simulink model "Battery_Pack_Thermal_Management"  (R2021b)
settings: Solver=ode23t  StartTime=0.0  StopTime=2400  MaxStep=0.05  RelTol=1e-3  AbsTol=1e-3
PreLoadFcn:
  | Battery_Pack_Thermal_Management_param
undefined symbols (not defined in the file): ambient, coolantTemp, R12, R23, R34, R45, R56, R67, R78
libraries: nesl_utility x35, fl_lib x10, batteryModule_lib x8, ee_lib x1
(part 1 of 2)
Description:
  | Battery Pack Thermal Management
  | 
  | Copyright 2020-2021 The MathWorks, Inc.
settings Model: Creator=vikrants  LastModifiedBy=smiller
settings SolverCC: AutoScaleAbsTol=off  AlgebraicLoopSolver=TrustRegion
settings DataIOCC: ReturnWorkspaceOutputs=off  SignalLoggingName=logsout_Battery_Pack_Thermal_Management
settings DebuggingCC: SymbolicDimsDataTypeCodeGenerationDiagnostic=none  SFMachineParentedDataDiag=warning
settings SFSimCC: CustomCodeUndefinedFunction=UseInterfaceOnly
settings SimscapeCC: SimscapeLogType=all  SimscapeLogSimulationStatistics=on  SimscapeLogName=simlog_Battery_Pack_Thermal_Management  SimscapeLogDataHistory=250000

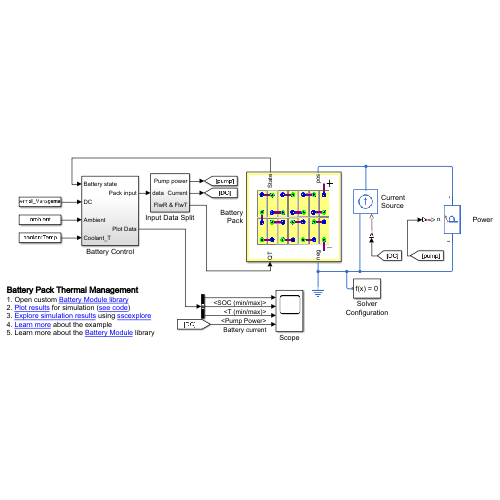
[thumbnail: Simulink's stored preview of the top-level diagram]
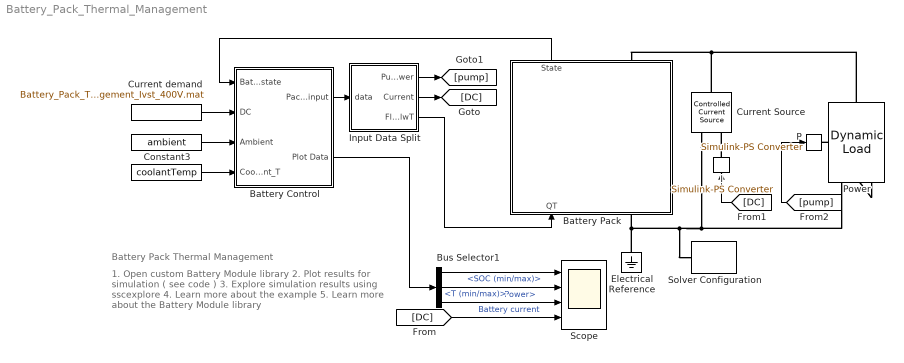
== system Battery_Pack_Thermal_Management ==
  note: 1. Open custom Battery Module library
      | 2. Plot results for simulation ( see code )
      | 3. Explore simulation results using sscexplore
      | 4. Learn more about the example
      | 5. Learn more about the Battery Module library
  note: Battery Pack Thermal Management
  " " : Constant  Value=coolantTemp
  Battery Pack : Subsystem
      mask Display: image('batteryPackIcon.png'); % Use "Edit Image" on toolstrip to change.
  Battery Control : Subsystem
  Bus Selector1 : BusSelector  OutputSignals=SOC (min/max),T (min/max),Pump Power
  Constant3 : Constant  Value=ambient
  Current Source : fl_lib/Electrical/Electrical Sources/Controlled Current Source
  Current demand : FromFile  FileName=Battery_Pack_Thermal_Management_Ivst_400V.mat  SampleTime=0
  Electrical Reference : fl_lib/Electrical/Electrical Elements/Electrical Reference
  I : nesl_utility/Simulink-PS Converter  PhysicalDomain=network_engine_domain  SubClassName=ps_input  LeftPortType=input  RightPortType=output  PseudoPeriodic=off  Frequencies=[]  NoiseDistribution=none  NoiseParameters=[]  Unit=A  AffineConversion=off  FilteringAndDerivatives=provide  SimscapeFilterOrder=1  InputFilterTimeConstant=0.001  UdotUserProvided=0
      settings: SourceProductName=Utilities
  Input Data Split : Subsystem
  P : nesl_utility/Simulink-PS Converter  PhysicalDomain=network_engine_domain  SubClassName=ps_input  LeftPortType=input  RightPortType=output  PseudoPeriodic=off  Frequencies=[]  NoiseDistribution=none  NoiseParameters=[]  Unit=J/s  AffineConversion=off  FilteringAndDerivatives=provide  SimscapeFilterOrder=1  InputFilterTimeConstant=0.001  UdotUserProvided=0
      settings: SourceProductName=Utilities
  Power : ee_lib/Passive/Dynamic Load  load_type=ee.enum.dc_ac.dc  min_supply_voltage=20 V  pow_min=1e-3 W  G_reverse=1e-6 S  deltaV=1e-3 V  f0=60 Hz  Vrms_min=200 V  Pmin=1e-3 W  enable_fault=simscape.enum.onoff.off  fault_action=simscape.enum.assert.action.none  t_fault=1 s  open_conductance=1e-4 S
      settings: SourceProductBaseCode=PS  InternalSimscapePortConfiguration="{\"Bottom\":[],\"Left\":[{\"id\":\"p\",\"label\":\"+\",\"type\":\"foundation.electrical.electrical\"}],\"Right\":[{\"id\":\"n\",\"label\":\"-\",\"type\":\"foundation.electrical.electrical\"}],\"Top\":[{\"id\":\"P\",\"label\":\"P\",\"type\":\"input\"}]}"
  Scope : Scope  NumInputPorts=4
  Solver Configuration : nesl_utility/Solver Configuration  PhysicalDomain=network_engine_domain  SubClassName=solver  LeftPortType=input  RightPortType=generic  Tones=[]  Harmonics=[]  SimulateNoise=off  Profile=off  UseLocalSampling=off  EnableSwitchedLinearOptims=on  FrequencyDomain=off  UseCCode=off  RelTol=0.001  AbsTol=1e-06  MinStep=1e-09  ToWorkspace=off  RevertToSquareIcSolve=off  NumHomotopyIterations=100  PhasorMode=off  PhasorModeNumHarmonics=1  DoDC=off  ResidualTolerance=1e-09  UseLocalSolver=off  LocalSolverChoice=NE_BACKWARD_EULER_ADVANCER  LocalSolverSampleTime=0.001  DoFixedCost=off  MaxNonlinIter=3  MaxModeIter=2  ComputeImpulses=off  ImpulseIterations=2  LinearAlgebra=auto  EquationFormulation=NE_TIME_EF  DelaysMemoryBudget=1024  AutomaticFiltering=on  FilteringTimeConstant=0.001  PartitionStorageMethod=AS_NEEDED  PartitionMemoryBudget=1024  PartitionMethod=ROBUST
      settings: SourceProductName=Utilities
  wires:
  Current demand/1 -> Battery Control/2(DC)
  Battery Pack/1(State) -> Battery Control/1(Battery state)
  Constant3/1 -> Battery Control/3(Ambient)
  Input Data Split/2(Current) -> [DC]
  Input Data Split/1(Pump power) -> [pump]
  [DC] -> Scope/4  "Battery current"
  Battery Control/1(Pack input) -> Input Data Split/1(data)
  Battery Control/2(Plot Data) -> Bus Selector1/1
  Bus Selector1/1 -> Scope/1  "<SOC (min/max)>"
  Bus Selector1/3 -> Scope/3  "<Pump Power>"
  Bus Selector1/2 -> Scope/2  "<T (min/max)>"
  Input Data Split/3(FlwR & FlwT) -> Battery Pack/1(QT)
  " "/1 -> Battery Control/4(Coolant_T)
  [DC] -> I/1
  [pump] -> P/1
  connections:
  Current Source/RConn2 -- Electrical Reference/LConn1 -- Battery Pack/LConn1 -- Solver Configuration/RConn1 -- Power/LConn1
  Current Source/LConn1 -- Power/RConn1 -- Battery Pack/RConn1
  Power/LConn2 -- P/RConn1
  I/RConn1 -- Current Source/RConn1

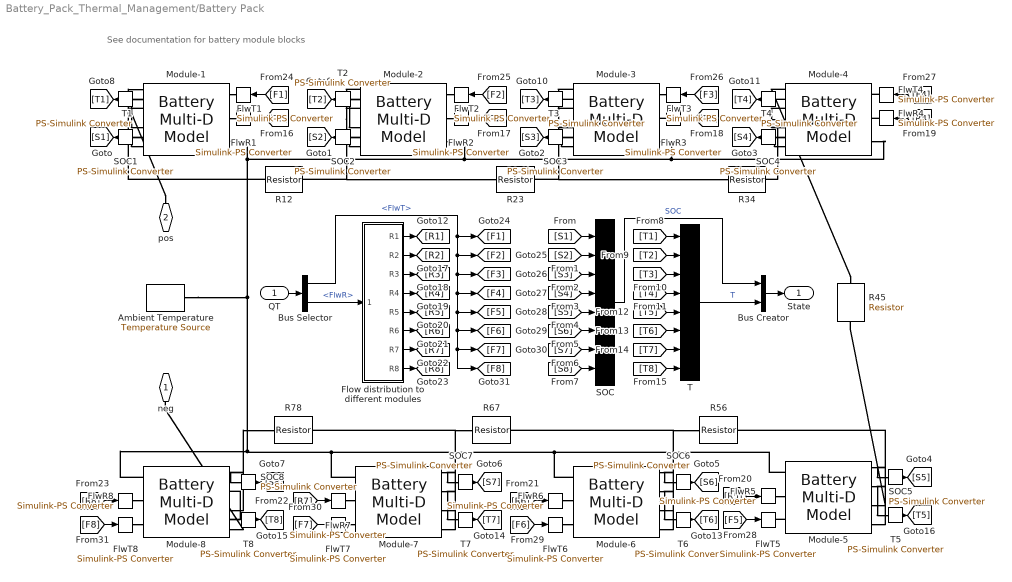
== system Battery_Pack_Thermal_Management/Battery Pack ==
  note: See documentation for battery module blocks
  QT : Inport
  Ambient Temperature : fl_lib/Thermal/Thermal Sources/Temperature Source  temperature=ambient K
  Bus Creator : BusCreator  Inputs=2
  Bus Selector : BusSelector  OutputSignals=FlwT,FlwR
  Flow distribution to different modules : Subsystem
  FlwR{1..8} (8 alike) : nesl_utility/Simulink-PS Converter  PhysicalDomain=network_engine_domain  SubClassName=ps_input  LeftPortType=input  RightPortType=output  PseudoPeriodic=off  Frequencies=[]  NoiseDistribution=none  NoiseParameters=[]  Unit=1  AffineConversion=off  FilteringAndDerivatives=provide  SimscapeFilterOrder=1  InputFilterTimeConstant=0.001  UdotUserProvided=0
      settings: SourceProductName=Utilities
  FlwT{1..8} (8 alike) : nesl_utility/Simulink-PS Converter  PhysicalDomain=network_engine_domain  SubClassName=ps_input  LeftPortType=input  RightPortType=output  PseudoPeriodic=off  Frequencies=[]  NoiseDistribution=none  NoiseParameters=[]  Unit=1  AffineConversion=off  FilteringAndDerivatives=provide  SimscapeFilterOrder=1  InputFilterTimeConstant=0.001  UdotUserProvided=0
      settings: SourceProductName=Utilities
  Module-1 : batteryModule_lib/Battery Multi-D Model  modelComplexity=batteryModule.batteryAbstractionLevel.grouped  LUTpointsTemp=T_vec K  cellAHvector=AH_vec hr*A  LUTpointsSOC=SOC_vec  V0_mat=V0_mat V  prm_dir=ee.enum.battery.prm_dir.noCurrentDirectionality  R0_mat=R0_mat Ohm  R0_dis_mat=[.03, .015, .002; .04, .017, .008; .039, .012, .006; .027, .013, .021] Ohm  R0_ch_mat=[.03, .015, .002; .04, .017, .008; .039, .012, .006; .027, .013, .021] Ohm  prm_leak=ee.enum.battery.prm_leak.disabled  Rleak_vec=[8000, 7000, 6000] Ohm  extrapolation_option=ee.enum.extrapolation.nearest  prm_dyn=ee.enum.battery.prm_dyn.rc2  R1_mat=R1_mat Ohm  tau1_mat=Tau1_mat s  R2_mat=R2_mat Ohm  tau2_mat=Tau2_mat s  R3_mat=[.014, .382, .407; .028, .006, .007; .014, .007, .006; .333, .956, .912] Ohm  tau3_mat=[1, 44, 5644; 11, 24, 506; 2, 14, 330; 3310, 13419, 30216] s  R4_mat=[.014, .382, .407; .028, .006, .007; .014, .007, .006; .333, .956, .912] Ohm  tau4_mat=[1, 44, 5644; 11, 24, 506; 2, 14, 330; 3310, 13419, 30216] s  R5_mat=[.014, .382, .407; .028, .006, .007; .014, .007, .006; .333, .956, .912] Ohm  tau5_mat=[1, 44, 5644; 11, 24, 506; 2, 14, 330; 3310, 13419, 30216] s  prm_fade=ee.enum.battery.prm_fade.equations  N0=Ndisc  dV0=delV0  dR0=delR0  dAH=delAH0  dRleak=0  dR1=delR1  dR2=delR2  dR3=0  dR4=0  dR5=0  N0vec=[100, 200, 300]  Tfadevec=[298.15, 323.15] K  dV0vec=[0, 0, 0]  dR0vec=[0, 0, 0]  dAHvec=[0, 0, 0]  dRleakvec=[0, 0, 0]  dR1vec=[0, 0, 0]  dR2vec=[0, 0, 0]  dR3vec=[0, 0, 0]  dR4vec=[0, 0, 0]  dR5vec=[0, 0, 0]  dV0mat=[0, 0; 0, 0; 0, 0]  dR0mat=[0, 0; 0, 0; 0, 0]  dAHmat=[0, 0; 0, 0; 0, 0]  dRleakmat=[0, 0; 0, 0; 0, 0]  dR1mat=[0, 0; 0, 0; 0, 0]  dR2mat=[0, 0; 0, 0; 0, 0]  dR3mat=[0, 0; 0, 0; 0, 0]  dR4mat=[0, 0; 0, 0; 0, 0]  dR5mat=[0, 0; 0, 0; 0, 0]  cellThermalMass=MdotCp J/K  cellThermalCond=K_cell W/(m*K)  cellThermalCond_inPlane=20 W/(m*K)  Ns=Ns1  Np=Np1  cellTypeSelection=batteryModule.batteryTypeSelection.pouch  cellHeight=cell_H m  cellWidth=cell_W m  cellThickness=cell_T m  cellDiameter=0.018 m  cellCylinLine=3  moduleExternalR=Rext1 Ohm  moduleCellBalancing=batteryModule.batteryCellBalancing.none  passiveShuntR=50 Ohm  passiveSWclosedR=0.01 Ohm  passiveSWopenCond=1e-8 1/Ohm  passiveSWthreshold=0.5  thermalManagement=batteryModule.batteryCoolingSystem.thermalPort  cellHeatTrCoeff=h_cell W/(m^2 * K)  thermal_moduleBottom=batteryModule.batteryThermalPortSelection.thermalLUT  htc_bottom=1 W/(m^2 * K)  moduleCooling_b=Q1 W/K  LUTpointsFlowrate_b=Flowrate_vec kg/s  LUTpointsTemp_b=T_vec K  thermal_moduleTop=batteryModule.batteryThermalPortSelection.convectionBC  htc_top=h_cell W/(m^2 * K)  moduleCooling_t=zeros(3, 6, 10) W/K  LUTpointsFlowrate_t=[.01, .02, .03, .04, .05, .06] kg/s  LUTpointsTemp_t=[273.15, 298.15, 323.15] K  thermal_moduleRight=batteryModule.batteryThermalPortSelection.convectionBC  htc_right=h_cell W/(m^2 * K)  moduleCooling_r=zeros(3, 6, 10) W/K  LUTpointsFlowrate_r=[.01, .02, .03, .04, .05, .06] kg/s  LUTpointsTemp_r=[273.15, 298.15, 323.15] K  thermal_moduleLeft=batteryModule.batteryThermalPortSelection.convectionBC  htc_left=h_cell W/(m^2 * K)  moduleCooling_l=zeros(3, 6, 10) W/K  LUTpointsFlowrate_l=[.01, .02, .03, .04, .05, .06] kg/s  LUTpointsTemp_l=[273.15, 298.15, 323.15] K  thermal_modulePos=batteryModule.batteryThermalPortSelection.convectionBC  htc_pos=h_cell W/(m^2 * K)  moduleCooling_p=zeros(3, 6, 10) W/K  LUTpointsFlowrate_p=[.01, .02, .03, .04, .05, .06] kg/s  LUTpointsTemp_p=[273.15, 298.15, 323.15] K  thermal_moduleNeg=batteryModule.batteryThermalPortSelection.convectionBC  htc_neg=h_cell W/(m^2 * K)  moduleCooling_n=zeros(3, 6, 10) W/K  LUTpointsFlowrate_n=[.01, .02, .03, .04, .05, .06] kg/s  LUTpointsTemp_n=[273.15, 298.15, 323.15] K  moduleExtHeat=extQ1 W  cellTemp=iniT1 K  cellSOC=iniSOC1  moduleCellAHpercentVar=iniAH1  moduleCellLeakPercentVar=ones(1, 10)  moduleCellR0PercentVar=iniR01
      settings: SourceProductName=Some kind of I/O error occurred when accessing database . (disk I/O error)  InternalSimscapePortConfiguration="{\"Bottom\":[],\"Left\":[{\"id\":\"outputCellSOC\",\"label\":\"SOC\",\"type\":\"output\"},{\"id\":\"outputCellTemp\",\"label\":\"Temp\",\"type\":\"output\"}],\"Right\":[{\"id\":\"H\",\"label\":\"Amb\",\"type\":\"foundation.thermal.thermal\"},{\"id\":\"frac_b\",\"label\":\"FlwR\",\"type\":\"input\"},{\"id\":\"delT_b\",\"label\":\"FlwT\",\"type\":\"input\"}],\"Top\":[{\"id\":\"p\",\"label\":\"pos\",\"type\":\"foundation.electrical.electrical\"},{\"id\":\"n\",\"label\":\"neg\",\"type\":\"foundation.electrical.electrical\"}]}"
  Module-2 : batteryModule_lib/Battery Multi-D Model  modelComplexity=batteryModule.batteryAbstractionLevel.grouped  LUTpointsTemp=T_vec K  cellAHvector=AH_vec hr*A  LUTpointsSOC=SOC_vec  V0_mat=V0_mat V  prm_dir=ee.enum.battery.prm_dir.noCurrentDirectionality  R0_mat=R0_mat Ohm  R0_dis_mat=[.03, .015, .002; .04, .017, .008; .039, .012, .006; .027, .013, .021] Ohm  R0_ch_mat=[.03, .015, .002; .04, .017, .008; .039, .012, .006; .027, .013, .021] Ohm  prm_leak=ee.enum.battery.prm_leak.disabled  Rleak_vec=[8000, 7000, 6000] Ohm  extrapolation_option=ee.enum.extrapolation.nearest  prm_dyn=ee.enum.battery.prm_dyn.rc2  R1_mat=R1_mat Ohm  tau1_mat=Tau1_mat s  R2_mat=R2_mat Ohm  tau2_mat=Tau2_mat s  R3_mat=[.014, .382, .407; .028, .006, .007; .014, .007, .006; .333, .956, .912] Ohm  tau3_mat=[1, 44, 5644; 11, 24, 506; 2, 14, 330; 3310, 13419, 30216] s  R4_mat=[.014, .382, .407; .028, .006, .007; .014, .007, .006; .333, .956, .912] Ohm  tau4_mat=[1, 44, 5644; 11, 24, 506; 2, 14, 330; 3310, 13419, 30216] s  R5_mat=[.014, .382, .407; .028, .006, .007; .014, .007, .006; .333, .956, .912] Ohm  tau5_mat=[1, 44, 5644; 11, 24, 506; 2, 14, 330; 3310, 13419, 30216] s  prm_fade=ee.enum.battery.prm_fade.equations  N0=Ndisc  dV0=delV0  dR0=delR0  dAH=delAH0  dRleak=0  dR1=delR1  dR2=delR2  dR3=0  dR4=0  dR5=0  N0vec=[100, 200, 300]  Tfadevec=[298.15, 323.15] K  dV0vec=[0, 0, 0]  dR0vec=[0, 0, 0]  dAHvec=[0, 0, 0]  dRleakvec=[0, 0, 0]  dR1vec=[0, 0, 0]  dR2vec=[0, 0, 0]  dR3vec=[0, 0, 0]  dR4vec=[0, 0, 0]  dR5vec=[0, 0, 0]  dV0mat=[0, 0; 0, 0; 0, 0]  dR0mat=[0, 0; 0, 0; 0, 0]  dAHmat=[0, 0; 0, 0; 0, 0]  dRleakmat=[0, 0; 0, 0; 0, 0]  dR1mat=[0, 0; 0, 0; 0, 0]  dR2mat=[0, 0; 0, 0; 0, 0]  dR3mat=[0, 0; 0, 0; 0, 0]  dR4mat=[0, 0; 0, 0; 0, 0]  dR5mat=[0, 0; 0, 0; 0, 0]  cellThermalMass=MdotCp J/K  cellThermalCond=K_cell W/(m*K)  cellThermalCond_inPlane=20 W/(m*K)  Ns=Ns2  Np=Np2  cellTypeSelection=batteryModule.batteryTypeSelection.pouch  cellHeight=cell_H m  cellWidth=cell_W m  cellThickness=cell_T m  cellDiameter=0.018 m  cellCylinLine=3  moduleExternalR=Rext2 Ohm  moduleCellBalancing=batteryModule.batteryCellBalancing.none  passiveShuntR=50 Ohm  passiveSWclosedR=0.01 Ohm  passiveSWopenCond=1e-8 1/Ohm  passiveSWthreshold=0.5  thermalManagement=batteryModule.batteryCoolingSystem.thermalPort  cellHeatTrCoeff=h_cell W/(m^2 * K)  thermal_moduleBottom=batteryModule.batteryThermalPortSelection.thermalLUT  htc_bottom=1 W/(m^2 * K)  moduleCooling_b=Q2 W/K  LUTpointsFlowrate_b=Flowrate_vec kg/s  LUTpointsTemp_b=T_vec K  thermal_moduleTop=batteryModule.batteryThermalPortSelection.convectionBC  htc_top=h_cell W/(m^2 * K)  moduleCooling_t=zeros(3, 6, 10) W/K  LUTpointsFlowrate_t=[.01, .02, .03, .04, .05, .06] kg/s  LUTpointsTemp_t=[273.15, 298.15, 323.15] K  thermal_moduleRight=batteryModule.batteryThermalPortSelection.convectionBC  htc_right=h_cell W/(m^2 * K)  moduleCooling_r=zeros(3, 6, 10) W/K  LUTpointsFlowrate_r=[.01, .02, .03, .04, .05, .06] kg/s  LUTpointsTemp_r=[273.15, 298.15, 323.15] K  thermal_moduleLeft=batteryModule.batteryThermalPortSelection.convectionBC  htc_left=h_cell W/(m^2 * K)  moduleCooling_l=zeros(3, 6, 10) W/K  LUTpointsFlowrate_l=[.01, .02, .03, .04, .05, .06] kg/s  LUTpointsTemp_l=[273.15, 298.15, 323.15] K  thermal_modulePos=batteryModule.batteryThermalPortSelection.convectionBC  htc_pos=h_cell W/(m^2 * K)  moduleCooling_p=zeros(3, 6, 10) W/K  LUTpointsFlowrate_p=[.01, .02, .03, .04, .05, .06] kg/s  LUTpointsTemp_p=[273.15, 298.15, 323.15] K  thermal_moduleNeg=batteryModule.batteryThermalPortSelection.convectionBC  htc_neg=h_cell W/(m^2 * K)  moduleCooling_n=zeros(3, 6, 10) W/K  LUTpointsFlowrate_n=[.01, .02, .03, .04, .05, .06] kg/s  LUTpointsTemp_n=[273.15, 298.15, 323.15] K  moduleExtHeat=extQ2 W  cellTemp=iniT2 K  cellSOC=iniSOC2  moduleCellAHpercentVar=iniAH2  moduleCellLeakPercentVar=ones(1, 10)  moduleCellR0PercentVar=iniR02
      settings: SourceProductName=Some kind of I/O error occurred when accessing database . (disk I/O error)  InternalSimscapePortConfiguration="{\"Bottom\":[],\"Left\":[{\"id\":\"outputCellSOC\",\"label\":\"SOC\",\"type\":\"output\"},{\"id\":\"outputCellTemp\",\"label\":\"Temp\",\"type\":\"output\"}],\"Right\":[{\"id\":\"H\",\"label\":\"Amb\",\"type\":\"foundation.thermal.thermal\"},{\"id\":\"frac_b\",\"label\":\"FlwR\",\"type\":\"input\"},{\"id\":\"delT_b\",\"label\":\"FlwT\",\"type\":\"input\"}],\"Top\":[{\"id\":\"p\",\"label\":\"pos\",\"type\":\"foundation.electrical.electrical\"},{\"id\":\"n\",\"label\":\"neg\",\"type\":\"foundation.electrical.electrical\"}]}"
  Module-3 : batteryModule_lib/Battery Multi-D Model  modelComplexity=batteryModule.batteryAbstractionLevel.grouped  LUTpointsTemp=T_vec K  cellAHvector=AH_vec hr*A  LUTpointsSOC=SOC_vec  V0_mat=V0_mat V  prm_dir=ee.enum.battery.prm_dir.noCurrentDirectionality  R0_mat=R0_mat Ohm  R0_dis_mat=[.03, .015, .002; .04, .017, .008; .039, .012, .006; .027, .013, .021] Ohm  R0_ch_mat=[.03, .015, .002; .04, .017, .008; .039, .012, .006; .027, .013, .021] Ohm  prm_leak=ee.enum.battery.prm_leak.disabled  Rleak_vec=[8000, 7000, 6000] Ohm  extrapolation_option=ee.enum.extrapolation.nearest  prm_dyn=ee.enum.battery.prm_dyn.rc2  R1_mat=R1_mat Ohm  tau1_mat=Tau1_mat s  R2_mat=R2_mat Ohm  tau2_mat=Tau2_mat s  R3_mat=[.014, .382, .407; .028, .006, .007; .014, .007, .006; .333, .956, .912] Ohm  tau3_mat=[1, 44, 5644; 11, 24, 506; 2, 14, 330; 3310, 13419, 30216] s  R4_mat=[.014, .382, .407; .028, .006, .007; .014, .007, .006; .333, .956, .912] Ohm  tau4_mat=[1, 44, 5644; 11, 24, 506; 2, 14, 330; 3310, 13419, 30216] s  R5_mat=[.014, .382, .407; .028, .006, .007; .014, .007, .006; .333, .956, .912] Ohm  tau5_mat=[1, 44, 5644; 11, 24, 506; 2, 14, 330; 3310, 13419, 30216] s  prm_fade=ee.enum.battery.prm_fade.equations  N0=Ndisc  dV0=delV0  dR0=delR0  dAH=delAH0  dRleak=0  dR1=delR1  dR2=delR2  dR3=0  dR4=0  dR5=0  N0vec=[100, 200, 300]  Tfadevec=[298.15, 323.15] K  dV0vec=[0, 0, 0]  dR0vec=[0, 0, 0]  dAHvec=[0, 0, 0]  dRleakvec=[0, 0, 0]  dR1vec=[0, 0, 0]  dR2vec=[0, 0, 0]  dR3vec=[0, 0, 0]  dR4vec=[0, 0, 0]  dR5vec=[0, 0, 0]  dV0mat=[0, 0; 0, 0; 0, 0]  dR0mat=[0, 0; 0, 0; 0, 0]  dAHmat=[0, 0; 0, 0; 0, 0]  dRleakmat=[0, 0; 0, 0; 0, 0]  dR1mat=[0, 0; 0, 0; 0, 0]  dR2mat=[0, 0; 0, 0; 0, 0]  dR3mat=[0, 0; 0, 0; 0, 0]  dR4mat=[0, 0; 0, 0; 0, 0]  dR5mat=[0, 0; 0, 0; 0, 0]  cellThermalMass=MdotCp J/K  cellThermalCond=K_cell W/(m*K)  cellThermalCond_inPlane=20 W/(m*K)  Ns=Ns3  Np=Np3  cellTypeSelection=batteryModule.batteryTypeSelection.pouch  cellHeight=cell_H m  cellWidth=cell_W m  cellThickness=cell_T m  cellDiameter=0.018 m  cellCylinLine=3  moduleExternalR=Rext3 Ohm  moduleCellBalancing=batteryModule.batteryCellBalancing.none  passiveShuntR=50 Ohm  passiveSWclosedR=0.01 Ohm  passiveSWopenCond=1e-8 1/Ohm  passiveSWthreshold=0.5  thermalManagement=batteryModule.batteryCoolingSystem.thermalPort  cellHeatTrCoeff=h_cell W/(m^2 * K)  thermal_moduleBottom=batteryModule.batteryThermalPortSelection.thermalLUT  htc_bottom=1 W/(m^2 * K)  moduleCooling_b=Q3 W/K  LUTpointsFlowrate_b=Flowrate_vec kg/s  LUTpointsTemp_b=T_vec K  thermal_moduleTop=batteryModule.batteryThermalPortSelection.convectionBC  htc_top=h_cell W/(m^2 * K)  moduleCooling_t=zeros(3, 6, 10) W/K  LUTpointsFlowrate_t=[.01, .02, .03, .04, .05, .06] kg/s  LUTpointsTemp_t=[273.15, 298.15, 323.15] K  thermal_moduleRight=batteryModule.batteryThermalPortSelection.convectionBC  htc_right=h_cell W/(m^2 * K)  moduleCooling_r=zeros(3, 6, 10) W/K  LUTpointsFlowrate_r=[.01, .02, .03, .04, .05, .06] kg/s  LUTpointsTemp_r=[273.15, 298.15, 323.15] K  thermal_moduleLeft=batteryModule.batteryThermalPortSelection.convectionBC  htc_left=h_cell W/(m^2 * K)  moduleCooling_l=zeros(3, 6, 10) W/K  LUTpointsFlowrate_l=[.01, .02, .03, .04, .05, .06] kg/s  LUTpointsTemp_l=[273.15, 298.15, 323.15] K  thermal_modulePos=batteryModule.batteryThermalPortSelection.convectionBC  htc_pos=h_cell W/(m^2 * K)  moduleCooling_p=zeros(3, 6, 10) W/K  LUTpointsFlowrate_p=[.01, .02, .03, .04, .05, .06] kg/s  LUTpointsTemp_p=[273.15, 298.15, 323.15] K  thermal_moduleNeg=batteryModule.batteryThermalPortSelection.convectionBC  htc_neg=h_cell W/(m^2 * K)  moduleCooling_n=zeros(3, 6, 10) W/K  LUTpointsFlowrate_n=[.01, .02, .03, .04, .05, .06] kg/s  LUTpointsTemp_n=[273.15, 298.15, 323.15] K  moduleExtHeat=extQ3 W  cellTemp=iniT3 K  cellSOC=iniSOC3  moduleCellAHpercentVar=iniAH3  moduleCellLeakPercentVar=ones(1, 10)  moduleCellR0PercentVar=iniR03
      settings: SourceProductName=Some kind of I/O error occurred when accessing database . (disk I/O error)  InternalSimscapePortConfiguration="{\"Bottom\":[],\"Left\":[{\"id\":\"outputCellSOC\",\"label\":\"SOC\",\"type\":\"output\"},{\"id\":\"outputCellTemp\",\"label\":\"Temp\",\"type\":\"output\"}],\"Right\":[{\"id\":\"H\",\"label\":\"Amb\",\"type\":\"foundation.thermal.thermal\"},{\"id\":\"frac_b\",\"label\":\"FlwR\",\"type\":\"input\"},{\"id\":\"delT_b\",\"label\":\"FlwT\",\"type\":\"input\"}],\"Top\":[{\"id\":\"p\",\"label\":\"pos\",\"type\":\"foundation.electrical.electrical\"},{\"id\":\"n\",\"label\":\"neg\",\"type\":\"foundation.electrical.electrical\"}]}"
  Module-4 : batteryModule_lib/Battery Multi-D Model  modelComplexity=batteryModule.batteryAbstractionLevel.grouped  LUTpointsTemp=T_vec K  cellAHvector=AH_vec hr*A  LUTpointsSOC=SOC_vec  V0_mat=V0_mat V  prm_dir=ee.enum.battery.prm_dir.noCurrentDirectionality  R0_mat=R0_mat Ohm  R0_dis_mat=[.03, .015, .002; .04, .017, .008; .039, .012, .006; .027, .013, .021] Ohm  R0_ch_mat=[.03, .015, .002; .04, .017, .008; .039, .012, .006; .027, .013, .021] Ohm  prm_leak=ee.enum.battery.prm_leak.disabled  Rleak_vec=[8000, 7000, 6000] Ohm  extrapolation_option=ee.enum.extrapolation.nearest  prm_dyn=ee.enum.battery.prm_dyn.rc2  R1_mat=R1_mat Ohm  tau1_mat=Tau1_mat s  R2_mat=R2_mat Ohm  tau2_mat=Tau2_mat s  R3_mat=[.014, .382, .407; .028, .006, .007; .014, .007, .006; .333, .956, .912] Ohm  tau3_mat=[1, 44, 5644; 11, 24, 506; 2, 14, 330; 3310, 13419, 30216] s  R4_mat=[.014, .382, .407; .028, .006, .007; .014, .007, .006; .333, .956, .912] Ohm  tau4_mat=[1, 44, 5644; 11, 24, 506; 2, 14, 330; 3310, 13419, 30216] s  R5_mat=[.014, .382, .407; .028, .006, .007; .014, .007, .006; .333, .956, .912] Ohm  tau5_mat=[1, 44, 5644; 11, 24, 506; 2, 14, 330; 3310, 13419, 30216] s  prm_fade=ee.enum.battery.prm_fade.equations  N0=Ndisc  dV0=delV0  dR0=delR0  dAH=delAH0  dRleak=0  dR1=delR1  dR2=delR2  dR3=0  dR4=0  dR5=0  N0vec=[100, 200, 300]  Tfadevec=[298.15, 323.15] K  dV0vec=[0, 0, 0]  dR0vec=[0, 0, 0]  dAHvec=[0, 0, 0]  dRleakvec=[0, 0, 0]  dR1vec=[0, 0, 0]  dR2vec=[0, 0, 0]  dR3vec=[0, 0, 0]  dR4vec=[0, 0, 0]  dR5vec=[0, 0, 0]  dV0mat=[0, 0; 0, 0; 0, 0]  dR0mat=[0, 0; 0, 0; 0, 0]  dAHmat=[0, 0; 0, 0; 0, 0]  dRleakmat=[0, 0; 0, 0; 0, 0]  dR1mat=[0, 0; 0, 0; 0, 0]  dR2mat=[0, 0; 0, 0; 0, 0]  dR3mat=[0, 0; 0, 0; 0, 0]  dR4mat=[0, 0; 0, 0; 0, 0]  dR5mat=[0, 0; 0, 0; 0, 0]  cellThermalMass=MdotCp J/K  cellThermalCond=K_cell W/(m*K)  cellThermalCond_inPlane=20 W/(m*K)  Ns=Ns4  Np=Np4  cellTypeSelection=batteryModule.batteryTypeSelection.pouch  cellHeight=cell_H m  cellWidth=cell_W m  cellThickness=cell_T m  cellDiameter=0.018 m  cellCylinLine=3  moduleExternalR=Rext4 Ohm  moduleCellBalancing=batteryModule.batteryCellBalancing.none  passiveShuntR=50 Ohm  passiveSWclosedR=0.01 Ohm  passiveSWopenCond=1e-8 1/Ohm  passiveSWthreshold=0.5  thermalManagement=batteryModule.batteryCoolingSystem.thermalPort  cellHeatTrCoeff=h_cell W/(m^2 * K)  thermal_moduleBottom=batteryModule.batteryThermalPortSelection.thermalLUT  htc_bottom=1 W/(m^2 * K)  moduleCooling_b=Q4 W/K  LUTpointsFlowrate_b=Flowrate_vec kg/s  LUTpointsTemp_b=T_vec K  thermal_moduleTop=batteryModule.batteryThermalPortSelection.convectionBC  htc_top=h_cell W/(m^2 * K)  moduleCooling_t=zeros(3, 6, 10) W/K  LUTpointsFlowrate_t=[.01, .02, .03, .04, .05, .06] kg/s  LUTpointsTemp_t=[273.15, 298.15, 323.15] K  thermal_moduleRight=batteryModule.batteryThermalPortSelection.convectionBC  htc_right=h_cell W/(m^2 * K)  moduleCooling_r=zeros(3, 6, 10) W/K  LUTpointsFlowrate_r=[.01, .02, .03, .04, .05, .06] kg/s  LUTpointsTemp_r=[273.15, 298.15, 323.15] K  thermal_moduleLeft=batteryModule.batteryThermalPortSelection.convectionBC  htc_left=h_cell W/(m^2 * K)  moduleCooling_l=zeros(3, 6, 10) W/K  LUTpointsFlowrate_l=[.01, .02, .03, .04, .05, .06] kg/s  LUTpointsTemp_l=[273.15, 298.15, 323.15] K  thermal_modulePos=batteryModule.batteryThermalPortSelection.convectionBC  htc_pos=h_cell W/(m^2 * K)  moduleCooling_p=zeros(3, 6, 10) W/K  LUTpointsFlowrate_p=[.01, .02, .03, .04, .05, .06] kg/s  LUTpointsTemp_p=[273.15, 298.15, 323.15] K  thermal_moduleNeg=batteryModule.batteryThermalPortSelection.convectionBC  htc_neg=h_cell W/(m^2 * K)  moduleCooling_n=zeros(3, 6, 10) W/K  LUTpointsFlowrate_n=[.01, .02, .03, .04, .05, .06] kg/s  LUTpointsTemp_n=[273.15, 298.15, 323.15] K  moduleExtHeat=extQ4 W  cellTemp=iniT4 K  cellSOC=iniSOC4  moduleCellAHpercentVar=iniAH4  moduleCellLeakPercentVar=ones(1, 10)  moduleCellR0PercentVar=iniR04
      settings: SourceProductName=Some kind of I/O error occurred when accessing database . (disk I/O error)  InternalSimscapePortConfiguration="{\"Bottom\":[],\"Left\":[{\"id\":\"outputCellSOC\",\"label\":\"SOC\",\"type\":\"output\"},{\"id\":\"outputCellTemp\",\"label\":\"Temp\",\"type\":\"output\"}],\"Right\":[{\"id\":\"H\",\"label\":\"Amb\",\"type\":\"foundation.thermal.thermal\"},{\"id\":\"frac_b\",\"label\":\"FlwR\",\"type\":\"input\"},{\"id\":\"delT_b\",\"label\":\"FlwT\",\"type\":\"input\"}],\"Top\":[{\"id\":\"p\",\"label\":\"pos\",\"type\":\"foundation.electrical.electrical\"},{\"id\":\"n\",\"label\":\"neg\",\"type\":\"foundation.electrical.electrical\"}]}"
  Module-5 : batteryModule_lib/Battery Multi-D Model  modelComplexity=batteryModule.batteryAbstractionLevel.grouped  LUTpointsTemp=T_vec K  cellAHvector=AH_vec hr*A  LUTpointsSOC=SOC_vec  V0_mat=V0_mat V  prm_dir=ee.enum.battery.prm_dir.noCurrentDirectionality  R0_mat=R0_mat Ohm  R0_dis_mat=[.03, .015, .002; .04, .017, .008; .039, .012, .006; .027, .013, .021] Ohm  R0_ch_mat=[.03, .015, .002; .04, .017, .008; .039, .012, .006; .027, .013, .021] Ohm  prm_leak=ee.enum.battery.prm_leak.disabled  Rleak_vec=[8000, 7000, 6000] Ohm  extrapolation_option=ee.enum.extrapolation.nearest  prm_dyn=ee.enum.battery.prm_dyn.rc2  R1_mat=R1_mat Ohm  tau1_mat=Tau1_mat s  R2_mat=R2_mat Ohm  tau2_mat=Tau2_mat s  R3_mat=[.014, .382, .407; .028, .006, .007; .014, .007, .006; .333, .956, .912] Ohm  tau3_mat=[1, 44, 5644; 11, 24, 506; 2, 14, 330; 3310, 13419, 30216] s  R4_mat=[.014, .382, .407; .028, .006, .007; .014, .007, .006; .333, .956, .912] Ohm  tau4_mat=[1, 44, 5644; 11, 24, 506; 2, 14, 330; 3310, 13419, 30216] s  R5_mat=[.014, .382, .407; .028, .006, .007; .014, .007, .006; .333, .956, .912] Ohm  tau5_mat=[1, 44, 5644; 11, 24, 506; 2, 14, 330; 3310, 13419, 30216] s  prm_fade=ee.enum.battery.prm_fade.equations  N0=Ndisc  dV0=delV0  dR0=delR0  dAH=delAH0  dRleak=0  dR1=delR1  dR2=delR2  dR3=0  dR4=0  dR5=0  N0vec=[100, 200, 300]  Tfadevec=[298.15, 323.15] K  dV0vec=[0, 0, 0]  dR0vec=[0, 0, 0]  dAHvec=[0, 0, 0]  dRleakvec=[0, 0, 0]  dR1vec=[0, 0, 0]  dR2vec=[0, 0, 0]  dR3vec=[0, 0, 0]  dR4vec=[0, 0, 0]  dR5vec=[0, 0, 0]  dV0mat=[0, 0; 0, 0; 0, 0]  dR0mat=[0, 0; 0, 0; 0, 0]  dAHmat=[0, 0; 0, 0; 0, 0]  dRleakmat=[0, 0; 0, 0; 0, 0]  dR1mat=[0, 0; 0, 0; 0, 0]  dR2mat=[0, 0; 0, 0; 0, 0]  dR3mat=[0, 0; 0, 0; 0, 0]  dR4mat=[0, 0; 0, 0; 0, 0]  dR5mat=[0, 0; 0, 0; 0, 0]  cellThermalMass=MdotCp J/K  cellThermalCond=K_cell W/(m*K)  cellThermalCond_inPlane=20 W/(m*K)  Ns=Ns5  Np=Np5  cellTypeSelection=batteryModule.batteryTypeSelection.pouch  cellHeight=cell_H m  cellWidth=cell_W m  cellThickness=cell_T m  cellDiameter=0.018 m  cellCylinLine=3  moduleExternalR=Rext5 Ohm  moduleCellBalancing=batteryModule.batteryCellBalancing.none  passiveShuntR=50 Ohm  passiveSWclosedR=0.01 Ohm  passiveSWopenCond=1e-8 1/Ohm  passiveSWthreshold=0.5  thermalManagement=batteryModule.batteryCoolingSystem.thermalPort  cellHeatTrCoeff=h_cell W/(m^2 * K)  thermal_moduleBottom=batteryModule.batteryThermalPortSelection.thermalLUT  htc_bottom=1 W/(m^2 * K)  moduleCooling_b=Q5 W/K  LUTpointsFlowrate_b=Flowrate_vec kg/s  LUTpointsTemp_b=T_vec K  thermal_moduleTop=batteryModule.batteryThermalPortSelection.convectionBC  htc_top=h_cell W/(m^2 * K)  moduleCooling_t=zeros(3, 6, 10) W/K  LUTpointsFlowrate_t=[.01, .02, .03, .04, .05, .06] kg/s  LUTpointsTemp_t=[273.15, 298.15, 323.15] K  thermal_moduleRight=batteryModule.batteryThermalPortSelection.convectionBC  htc_right=h_cell W/(m^2 * K)  moduleCooling_r=zeros(3, 6, 10) W/K  LUTpointsFlowrate_r=[.01, .02, .03, .04, .05, .06] kg/s  LUTpointsTemp_r=[273.15, 298.15, 323.15] K  thermal_moduleLeft=batteryModule.batteryThermalPortSelection.convectionBC  htc_left=h_cell W/(m^2 * K)  moduleCooling_l=zeros(3, 6, 10) W/K  LUTpointsFlowrate_l=[.01, .02, .03, .04, .05, .06] kg/s  LUTpointsTemp_l=[273.15, 298.15, 323.15] K  thermal_modulePos=batteryModule.batteryThermalPortSelection.convectionBC  htc_pos=h_cell W/(m^2 * K)  moduleCooling_p=zeros(3, 6, 10) W/K  LUTpointsFlowrate_p=[.01, .02, .03, .04, .05, .06] kg/s  LUTpointsTemp_p=[273.15, 298.15, 323.15] K  thermal_moduleNeg=batteryModule.batteryThermalPortSelection.convectionBC  htc_neg=h_cell W/(m^2 * K)  moduleCooling_n=zeros(3, 6, 10) W/K  LUTpointsFlowrate_n=[.01, .02, .03, .04, .05, .06] kg/s  LUTpointsTemp_n=[273.15, 298.15, 323.15] K  moduleExtHeat=extQ5 W  cellTemp=iniT5 K  cellSOC=iniSOC5  moduleCellAHpercentVar=iniAH5  moduleCellLeakPercentVar=ones(1, 10)  moduleCellR0PercentVar=iniR05
      settings: SourceProductName=Some kind of I/O error occurred when accessing database . (disk I/O error)  InternalSimscapePortConfiguration="{\"Bottom\":[],\"Left\":[{\"id\":\"outputCellSOC\",\"label\":\"SOC\",\"type\":\"output\"},{\"id\":\"outputCellTemp\",\"label\":\"Temp\",\"type\":\"output\"}],\"Right\":[{\"id\":\"H\",\"label\":\"Amb\",\"type\":\"foundation.thermal.thermal\"},{\"id\":\"frac_b\",\"label\":\"FlwR\",\"type\":\"input\"},{\"id\":\"delT_b\",\"label\":\"FlwT\",\"type\":\"input\"}],\"Top\":[{\"id\":\"p\",\"label\":\"pos\",\"type\":\"foundation.electrical.electrical\"},{\"id\":\"n\",\"label\":\"neg\",\"type\":\"foundation.electrical.electrical\"}]}"
  Module-6 : batteryModule_lib/Battery Multi-D Model  modelComplexity=batteryModule.batteryAbstractionLevel.grouped  LUTpointsTemp=T_vec K  cellAHvector=AH_vec hr*A  LUTpointsSOC=SOC_vec  V0_mat=V0_mat V  prm_dir=ee.enum.battery.prm_dir.noCurrentDirectionality  R0_mat=R0_mat Ohm  R0_dis_mat=[.03, .015, .002; .04, .017, .008; .039, .012, .006; .027, .013, .021] Ohm  R0_ch_mat=[.03, .015, .002; .04, .017, .008; .039, .012, .006; .027, .013, .021] Ohm  prm_leak=ee.enum.battery.prm_leak.disabled  Rleak_vec=[8000, 7000, 6000] Ohm  extrapolation_option=ee.enum.extrapolation.nearest  prm_dyn=ee.enum.battery.prm_dyn.rc2  R1_mat=R1_mat Ohm  tau1_mat=Tau1_mat s  R2_mat=R2_mat Ohm  tau2_mat=Tau2_mat s  R3_mat=[.014, .382, .407; .028, .006, .007; .014, .007, .006; .333, .956, .912] Ohm  tau3_mat=[1, 44, 5644; 11, 24, 506; 2, 14, 330; 3310, 13419, 30216] s  R4_mat=[.014, .382, .407; .028, .006, .007; .014, .007, .006; .333, .956, .912] Ohm  tau4_mat=[1, 44, 5644; 11, 24, 506; 2, 14, 330; 3310, 13419, 30216] s  R5_mat=[.014, .382, .407; .028, .006, .007; .014, .007, .006; .333, .956, .912] Ohm  tau5_mat=[1, 44, 5644; 11, 24, 506; 2, 14, 330; 3310, 13419, 30216] s  prm_fade=ee.enum.battery.prm_fade.equations  N0=Ndisc  dV0=delV0  dR0=delR0  dAH=delAH0  dRleak=0  dR1=delR1  dR2=delR2  dR3=0  dR4=0  dR5=0  N0vec=[100, 200, 300]  Tfadevec=[298.15, 323.15] K  dV0vec=[0, 0, 0]  dR0vec=[0, 0, 0]  dAHvec=[0, 0, 0]  dRleakvec=[0, 0, 0]  dR1vec=[0, 0, 0]  dR2vec=[0, 0, 0]  dR3vec=[0, 0, 0]  dR4vec=[0, 0, 0]  dR5vec=[0, 0, 0]  dV0mat=[0, 0; 0, 0; 0, 0]  dR0mat=[0, 0; 0, 0; 0, 0]  dAHmat=[0, 0; 0, 0; 0, 0]  dRleakmat=[0, 0; 0, 0; 0, 0]  dR1mat=[0, 0; 0, 0; 0, 0]  dR2mat=[0, 0; 0, 0; 0, 0]  dR3mat=[0, 0; 0, 0; 0, 0]  dR4mat=[0, 0; 0, 0; 0, 0]  dR5mat=[0, 0; 0, 0; 0, 0]  cellThermalMass=MdotCp J/K  cellThermalCond=K_cell W/(m*K)  cellThermalCond_inPlane=20 W/(m*K)  Ns=Ns6  Np=Np6  cellTypeSelection=batteryModule.batteryTypeSelection.pouch  cellHeight=cell_H m  cellWidth=cell_W m  cellThickness=cell_T m  cellDiameter=0.018 m  cellCylinLine=3  moduleExternalR=Rext6 Ohm  moduleCellBalancing=batteryModule.batteryCellBalancing.none  passiveShuntR=50 Ohm  passiveSWclosedR=0.01 Ohm  passiveSWopenCond=1e-8 1/Ohm  passiveSWthreshold=0.5  thermalManagement=batteryModule.batteryCoolingSystem.thermalPort  cellHeatTrCoeff=h_cell W/(m^2 * K)  thermal_moduleBottom=batteryModule.batteryThermalPortSelection.thermalLUT  htc_bottom=1 W/(m^2 * K)  moduleCooling_b=Q6 W/K  LUTpointsFlowrate_b=Flowrate_vec kg/s  LUTpointsTemp_b=T_vec K  thermal_moduleTop=batteryModule.batteryThermalPortSelection.convectionBC  htc_top=h_cell W/(m^2 * K)  moduleCooling_t=zeros(3, 6, 10) W/K  LUTpointsFlowrate_t=[.01, .02, .03, .04, .05, .06] kg/s  LUTpointsTemp_t=[273.15, 298.15, 323.15] K  thermal_moduleRight=batteryModule.batteryThermalPortSelection.convectionBC  htc_right=h_cell W/(m^2 * K)  moduleCooling_r=zeros(3, 6, 10) W/K  LUTpointsFlowrate_r=[.01, .02, .03, .04, .05, .06] kg/s  LUTpointsTemp_r=[273.15, 298.15, 323.15] K  thermal_moduleLeft=batteryModule.batteryThermalPortSelection.convectionBC  htc_left=h_cell W/(m^2 * K)  moduleCooling_l=zeros(3, 6, 10) W/K  LUTpointsFlowrate_l=[.01, .02, .03, .04, .05, .06] kg/s  LUTpointsTemp_l=[273.15, 298.15, 323.15] K  thermal_modulePos=batteryModule.batteryThermalPortSelection.convectionBC  htc_pos=h_cell W/(m^2 * K)  moduleCooling_p=zeros(3, 6, 10) W/K  LUTpointsFlowrate_p=[.01, .02, .03, .04, .05, .06] kg/s  LUTpointsTemp_p=[273.15, 298.15, 323.15] K  thermal_moduleNeg=batteryModule.batteryThermalPortSelection.convectionBC  htc_neg=h_cell W/(m^2 * K)  moduleCooling_n=zeros(3, 6, 10) W/K  LUTpointsFlowrate_n=[.01, .02, .03, .04, .05, .06] kg/s  LUTpointsTemp_n=[273.15, 298.15, 323.15] K  moduleExtHeat=extQ6 W  cellTemp=iniT6 K  cellSOC=iniSOC6  moduleCellAHpercentVar=iniAH6  moduleCellLeakPercentVar=ones(1, 10)  moduleCellR0PercentVar=iniR06
      settings: SourceProductName=Some kind of I/O error occurred when accessing database . (disk I/O error)  InternalSimscapePortConfiguration="{\"Bottom\":[],\"Left\":[{\"id\":\"outputCellSOC\",\"label\":\"SOC\",\"type\":\"output\"},{\"id\":\"outputCellTemp\",\"label\":\"Temp\",\"type\":\"output\"}],\"Right\":[{\"id\":\"H\",\"label\":\"Amb\",\"type\":\"foundation.thermal.thermal\"},{\"id\":\"frac_b\",\"label\":\"FlwR\",\"type\":\"input\"},{\"id\":\"delT_b\",\"label\":\"FlwT\",\"type\":\"input\"}],\"Top\":[{\"id\":\"p\",\"label\":\"pos\",\"type\":\"foundation.electrical.electrical\"},{\"id\":\"n\",\"label\":\"neg\",\"type\":\"foundation.electrical.electrical\"}]}"
  Module-7 : batteryModule_lib/Battery Multi-D Model  modelComplexity=batteryModule.batteryAbstractionLevel.grouped  LUTpointsTemp=T_vec K  cellAHvector=AH_vec hr*A  LUTpointsSOC=SOC_vec  V0_mat=V0_mat V  prm_dir=ee.enum.battery.prm_dir.noCurrentDirectionality  R0_mat=R0_mat Ohm  R0_dis_mat=[.03, .015, .002; .04, .017, .008; .039, .012, .006; .027, .013, .021] Ohm  R0_ch_mat=[.03, .015, .002; .04, .017, .008; .039, .012, .006; .027, .013, .021] Ohm  prm_leak=ee.enum.battery.prm_leak.disabled  Rleak_vec=[8000, 7000, 6000] Ohm  extrapolation_option=ee.enum.extrapolation.nearest  prm_dyn=ee.enum.battery.prm_dyn.rc2  R1_mat=R1_mat Ohm  tau1_mat=Tau1_mat s  R2_mat=R2_mat Ohm  tau2_mat=Tau2_mat s  R3_mat=[.014, .382, .407; .028, .006, .007; .014, .007, .006; .333, .956, .912] Ohm  tau3_mat=[1, 44, 5644; 11, 24, 506; 2, 14, 330; 3310, 13419, 30216] s  R4_mat=[.014, .382, .407; .028, .006, .007; .014, .007, .006; .333, .956, .912] Ohm  tau4_mat=[1, 44, 5644; 11, 24, 506; 2, 14, 330; 3310, 13419, 30216] s  R5_mat=[.014, .382, .407; .028, .006, .007; .014, .007, .006; .333, .956, .912] Ohm  tau5_mat=[1, 44, 5644; 11, 24, 506; 2, 14, 330; 3310, 13419, 30216] s  prm_fade=ee.enum.battery.prm_fade.equations  N0=Ndisc  dV0=delV0  dR0=delR0  dAH=delAH0  dRleak=0  dR1=delR1  dR2=delR2  dR3=0  dR4=0  dR5=0  N0vec=[100, 200, 300]  Tfadevec=[298.15, 323.15] K  dV0vec=[0, 0, 0]  dR0vec=[0, 0, 0]  dAHvec=[0, 0, 0]  dRleakvec=[0, 0, 0]  dR1vec=[0, 0, 0]  dR2vec=[0, 0, 0]  dR3vec=[0, 0, 0]  dR4vec=[0, 0, 0]  dR5vec=[0, 0, 0]  dV0mat=[0, 0; 0, 0; 0, 0]  dR0mat=[0, 0; 0, 0; 0, 0]  dAHmat=[0, 0; 0, 0; 0, 0]  dRleakmat=[0, 0; 0, 0; 0, 0]  dR1mat=[0, 0; 0, 0; 0, 0]  dR2mat=[0, 0; 0, 0; 0, 0]  dR3mat=[0, 0; 0, 0; 0, 0]  dR4mat=[0, 0; 0, 0; 0, 0]  dR5mat=[0, 0; 0, 0; 0, 0]  cellThermalMass=MdotCp J/K  cellThermalCond=K_cell W/(m*K)  cellThermalCond_inPlane=20 W/(m*K)  Ns=Ns7  Np=Np7  cellTypeSelection=batteryModule.batteryTypeSelection.pouch  cellHeight=cell_H m  cellWidth=cell_W m  cellThickness=cell_T m  cellDiameter=0.018 m  cellCylinLine=3  moduleExternalR=Rext7 Ohm  moduleCellBalancing=batteryModule.batteryCellBalancing.none  passiveShuntR=50 Ohm  passiveSWclosedR=0.01 Ohm  passiveSWopenCond=1e-8 1/Ohm  passiveSWthreshold=0.5  thermalManagement=batteryModule.batteryCoolingSystem.thermalPort  cellHeatTrCoeff=h_cell W/(m^2 * K)  thermal_moduleBottom=batteryModule.batteryThermalPortSelection.thermalLUT  htc_bottom=1 W/(m^2 * K)  moduleCooling_b=Q7 W/K  LUTpointsFlowrate_b=Flowrate_vec kg/s  LUTpointsTemp_b=T_vec K  thermal_moduleTop=batteryModule.batteryThermalPortSelection.convectionBC  htc_top=h_cell W/(m^2 * K)  moduleCooling_t=zeros(3, 6, 10) W/K  LUTpointsFlowrate_t=[.01, .02, .03, .04, .05, .06] kg/s  LUTpointsTemp_t=[273.15, 298.15, 323.15] K  thermal_moduleRight=batteryModule.batteryThermalPortSelection.convectionBC  htc_right=h_cell W/(m^2 * K)  moduleCooling_r=zeros(3, 6, 10) W/K  LUTpointsFlowrate_r=[.01, .02, .03, .04, .05, .06] kg/s  LUTpointsTemp_r=[273.15, 298.15, 323.15] K  thermal_moduleLeft=batteryModule.batteryThermalPortSelection.convectionBC  htc_left=h_cell W/(m^2 * K)  moduleCooling_l=zeros(3, 6, 10) W/K  LUTpointsFlowrate_l=[.01, .02, .03, .04, .05, .06] kg/s  LUTpointsTemp_l=[273.15, 298.15, 323.15] K  thermal_modulePos=batteryModule.batteryThermalPortSelection.convectionBC  htc_pos=h_cell W/(m^2 * K)  moduleCooling_p=zeros(3, 6, 10) W/K  LUTpointsFlowrate_p=[.01, .02, .03, .04, .05, .06] kg/s  LUTpointsTemp_p=[273.15, 298.15, 323.15] K  thermal_moduleNeg=batteryModule.batteryThermalPortSelection.convectionBC  htc_neg=h_cell W/(m^2 * K)  moduleCooling_n=zeros(3, 6, 10) W/K  LUTpointsFlowrate_n=[.01, .02, .03, .04, .05, .06] kg/s  LUTpointsTemp_n=[273.15, 298.15, 323.15] K  moduleExtHeat=extQ7 W  cellTemp=iniT7 K  cellSOC=iniSOC7  moduleCellAHpercentVar=iniAH7  moduleCellLeakPercentVar=ones(1, 10)  moduleCellR0PercentVar=iniR07
      settings: SourceProductName=Some kind of I/O error occurred when accessing database . (disk I/O error)  InternalSimscapePortConfiguration="{\"Bottom\":[],\"Left\":[{\"id\":\"outputCellSOC\",\"label\":\"SOC\",\"type\":\"output\"},{\"id\":\"outputCellTemp\",\"label\":\"Temp\",\"type\":\"output\"}],\"Right\":[{\"id\":\"H\",\"label\":\"Amb\",\"type\":\"foundation.thermal.thermal\"},{\"id\":\"frac_b\",\"label\":\"FlwR\",\"type\":\"input\"},{\"id\":\"delT_b\",\"label\":\"FlwT\",\"type\":\"input\"}],\"Top\":[{\"id\":\"p\",\"label\":\"pos\",\"type\":\"foundation.electrical.electrical\"},{\"id\":\"n\",\"label\":\"neg\",\"type\":\"foundation.electrical.electrical\"}]}"
  Module-8 : batteryModule_lib/Battery Multi-D Model  modelComplexity=batteryModule.batteryAbstractionLevel.grouped  LUTpointsTemp=T_vec K  cellAHvector=AH_vec hr*A  LUTpointsSOC=SOC_vec  V0_mat=V0_mat V  prm_dir=ee.enum.battery.prm_dir.noCurrentDirectionality  R0_mat=R0_mat Ohm  R0_dis_mat=[.03, .015, .002; .04, .017, .008; .039, .012, .006; .027, .013, .021] Ohm  R0_ch_mat=[.03, .015, .002; .04, .017, .008; .039, .012, .006; .027, .013, .021] Ohm  prm_leak=ee.enum.battery.prm_leak.disabled  Rleak_vec=[8000, 7000, 6000] Ohm  extrapolation_option=ee.enum.extrapolation.nearest  prm_dyn=ee.enum.battery.prm_dyn.rc2  R1_mat=R1_mat Ohm  tau1_mat=Tau1_mat s  R2_mat=R2_mat Ohm  tau2_mat=Tau2_mat s  R3_mat=[.014, .382, .407; .028, .006, .007; .014, .007, .006; .333, .956, .912] Ohm  tau3_mat=[1, 44, 5644; 11, 24, 506; 2, 14, 330; 3310, 13419, 30216] s  R4_mat=[.014, .382, .407; .028, .006, .007; .014, .007, .006; .333, .956, .912] Ohm  tau4_mat=[1, 44, 5644; 11, 24, 506; 2, 14, 330; 3310, 13419, 30216] s  R5_mat=[.014, .382, .407; .028, .006, .007; .014, .007, .006; .333, .956, .912] Ohm  tau5_mat=[1, 44, 5644; 11, 24, 506; 2, 14, 330; 3310, 13419, 30216] s  prm_fade=ee.enum.battery.prm_fade.equations  N0=Ndisc  dV0=delV0  dR0=delR0  dAH=delAH0  dRleak=0  dR1=delR1  dR2=delR2  dR3=0  dR4=0  dR5=0  N0vec=[100, 200, 300]  Tfadevec=[298.15, 323.15] K  dV0vec=[0, 0, 0]  dR0vec=[0, 0, 0]  dAHvec=[0, 0, 0]  dRleakvec=[0, 0, 0]  dR1vec=[0, 0, 0]  dR2vec=[0, 0, 0]  dR3vec=[0, 0, 0]  dR4vec=[0, 0, 0]  dR5vec=[0, 0, 0]  dV0mat=[0, 0; 0, 0; 0, 0]  dR0mat=[0, 0; 0, 0; 0, 0]  dAHmat=[0, 0; 0, 0; 0, 0]  dRleakmat=[0, 0; 0, 0; 0, 0]  dR1mat=[0, 0; 0, 0; 0, 0]  dR2mat=[0, 0; 0, 0; 0, 0]  dR3mat=[0, 0; 0, 0; 0, 0]  dR4mat=[0, 0; 0, 0; 0, 0]  dR5mat=[0, 0; 0, 0; 0, 0]  cellThermalMass=MdotCp J/K  cellThermalCond=K_cell W/(m*K)  cellThermalCond_inPlane=20 W/(m*K)  Ns=Ns8  Np=Np8  cellTypeSelection=batteryModule.batteryTypeSelection.pouch  cellHeight=cell_H m  cellWidth=cell_W m  cellThickness=cell_T m  cellDiameter=0.018 m  cellCylinLine=3  moduleExternalR=Rext8 Ohm  moduleCellBalancing=batteryModule.batteryCellBalancing.none  passiveShuntR=50 Ohm  passiveSWclosedR=0.01 Ohm  passiveSWopenCond=1e-8 1/Ohm  passiveSWthreshold=0.5  thermalManagement=batteryModule.batteryCoolingSystem.thermalPort  cellHeatTrCoeff=h_cell W/(m^2 * K)  thermal_moduleBottom=batteryModule.batteryThermalPortSelection.thermalLUT  htc_bottom=1 W/(m^2 * K)  moduleCooling_b=Q8 W/K  LUTpointsFlowrate_b=Flowrate_vec kg/s  LUTpointsTemp_b=T_vec K  thermal_moduleTop=batteryModule.batteryThermalPortSelection.convectionBC  htc_top=h_cell W/(m^2 * K)  moduleCooling_t=zeros(3, 6, 10) W/K  LUTpointsFlowrate_t=[.01, .02, .03, .04, .05, .06] kg/s  LUTpointsTemp_t=[273.15, 298.15, 323.15] K  thermal_moduleRight=batteryModule.batteryThermalPortSelection.convectionBC  htc_right=h_cell W/(m^2 * K)  moduleCooling_r=zeros(3, 6, 10) W/K  LUTpointsFlowrate_r=[.01, .02, .03, .04, .05, .06] kg/s  LUTpointsTemp_r=[273.15, 298.15, 323.15] K  thermal_moduleLeft=batteryModule.batteryThermalPortSelection.convectionBC  htc_left=h_cell W/(m^2 * K)  moduleCooling_l=zeros(3, 6, 10) W/K  LUTpointsFlowrate_l=[.01, .02, .03, .04, .05, .06] kg/s  LUTpointsTemp_l=[273.15, 298.15, 323.15] K  thermal_modulePos=batteryModule.batteryThermalPortSelection.convectionBC  htc_pos=h_cell W/(m^2 * K)  moduleCooling_p=zeros(3, 6, 10) W/K  LUTpointsFlowrate_p=[.01, .02, .03, .04, .05, .06] kg/s  LUTpointsTemp_p=[273.15, 298.15, 323.15] K  thermal_moduleNeg=batteryModule.batteryThermalPortSelection.convectionBC  htc_neg=h_cell W/(m^2 * K)  moduleCooling_n=zeros(3, 6, 10) W/K  LUTpointsFlowrate_n=[.01, .02, .03, .04, .05, .06] kg/s  LUTpointsTemp_n=[273.15, 298.15, 323.15] K  moduleExtHeat=extQ8 W  cellTemp=iniT8 K  cellSOC=iniSOC8  moduleCellAHpercentVar=iniAH8  moduleCellLeakPercentVar=ones(1, 10)  moduleCellR0PercentVar=iniR08
      settings: SourceProductName=Some kind of I/O error occurred when accessing database . (disk I/O error)  InternalSimscapePortConfiguration="{\"Bottom\":[],\"Left\":[{\"id\":\"outputCellSOC\",\"label\":\"SOC\",\"type\":\"output\"},{\"id\":\"outputCellTemp\",\"label\":\"Temp\",\"type\":\"output\"}],\"Right\":[{\"id\":\"H\",\"label\":\"Amb\",\"type\":\"foundation.thermal.thermal\"},{\"id\":\"frac_b\",\"label\":\"FlwR\",\"type\":\"input\"},{\"id\":\"delT_b\",\"label\":\"FlwT\",\"type\":\"input\"}],\"Top\":[{\"id\":\"p\",\"label\":\"pos\",\"type\":\"foundation.electrical.electrical\"},{\"id\":\"n\",\"label\":\"neg\",\"type\":\"foundation.electrical.electrical\"}]}"
  R12 : fl_lib/Electrical/Electrical Elements/Resistor  R=R12 Ohm  i_specify=off  i_priority=None  i=0 A  i_nominal_specify=off  i_nominal_unit=A  i_nominal_value=1  v_specify=off  v_priority=None  v=0 V  v_nominal_specify=off  v_nominal_unit=V  v_nominal_value=1
  R23 : fl_lib/Electrical/Electrical Elements/Resistor  R=R23 Ohm  i_specify=off  i_priority=None  i=0 A  i_nominal_specify=off  i_nominal_unit=A  i_nominal_value=1  v_specify=off  v_priority=None  v=0 V  v_nominal_specify=off  v_nominal_unit=V  v_nominal_value=1
  R34 : fl_lib/Electrical/Electrical Elements/Resistor  R=R34 Ohm  i_specify=off  i_priority=None  i=0 A  i_nominal_specify=off  i_nominal_unit=A  i_nominal_value=1  v_specify=off  v_priority=None  v=0 V  v_nominal_specify=off  v_nominal_unit=V  v_nominal_value=1
  R45 : fl_lib/Electrical/Electrical Elements/Resistor  R=R45 Ohm  i_specify=off  i_priority=None  i=0 A  i_nominal_specify=off  i_nominal_unit=A  i_nominal_value=1  v_specify=off  v_priority=None  v=0 V  v_nominal_specify=off  v_nominal_unit=V  v_nominal_value=1
  R56 : fl_lib/Electrical/Electrical Elements/Resistor  R=R56 Ohm  i_specify=off  i_priority=None  i=0 A  i_nominal_specify=off  i_nominal_unit=A  i_nominal_value=1  v_specify=off  v_priority=None  v=0 V  v_nominal_specify=off  v_nominal_unit=V  v_nominal_value=1
  R67 : fl_lib/Electrical/Electrical Elements/Resistor  R=R67 Ohm  i_specify=off  i_priority=None  i=0 A  i_nominal_specify=off  i_nominal_unit=A  i_nominal_value=1  v_specify=off  v_priority=None  v=0 V  v_nominal_specify=off  v_nominal_unit=V  v_nominal_value=1
  R78 : fl_lib/Electrical/Electrical Elements/Resistor  R=R78 Ohm  i_specify=off  i_priority=None  i=0 A  i_nominal_specify=off  i_nominal_unit=A  i_nominal_value=1  v_specify=off  v_priority=None  v=0 V  v_nominal_specify=off  v_nominal_unit=V  v_nominal_value=1
  SOC : Concatenate  NumInputs=8
  SOC{1..8} (8 alike) : nesl_utility/PS-Simulink Converter  PhysicalDomain=network_engine_domain  SubClassName=ps_output  LeftPortType=input  RightPortType=output  PseudoPeriodic=off  Frequencies=[]  Unit=inherit  AffineConversion=off
      settings: SourceProductName=Utilities
  T : Concatenate  NumInputs=8
  T{1..8} (8 alike) : nesl_utility/PS-Simulink Converter  PhysicalDomain=network_engine_domain  SubClassName=ps_output  LeftPortType=input  RightPortType=output  PseudoPeriodic=off  Frequencies=[]  Unit=inherit  AffineConversion=off
      settings: SourceProductName=Utilities
  neg : PMIOPort  Side=Left
  pos : PMIOPort  Port=2  Side=Right
  State : Outport
  wires:
  SOC7/1 -> [S7]
  [T3] -> T/3
  [R4] -> FlwR4/1
  [R6] -> FlwR6/1
  T5/1 -> [T5]
  [S7] -> SOC/7
  [S6] -> SOC/6
  [S8] -> SOC/8
  T8/1 -> [T8]
  [T1] -> T/1
  [S3] -> SOC/3
  [F4] -> FlwT4/1
  SOC2/1 -> [S2]
  [T4] -> T/4
  [R2] -> FlwR2/1
  [F5] -> FlwT5/1
  [R7] -> FlwR7/1
  SOC1/1 -> [S1]
  [T5] -> T/5
  SOC5/1 -> [S5]
  T3/1 -> [T3]
  [F2] -> FlwT2/1
  [T6] -> T/6
  T2/1 -> [T2]
  T7/1 -> [T7]
  [S1] -> SOC/1
  [S5] -> SOC/5
  T1/1 -> [T1]
  [T2] -> T/2
  [S4] -> SOC/4
  [R8] -> FlwR8/1
  T/1 -> Bus Creator/2  "T"
  [S2] -> SOC/2
  [F8] -> FlwT8/1
  [R3] -> FlwR3/1
  [T8] -> T/8
  SOC3/1 -> [S3]
  SOC4/1 -> [S4]
  [F3] -> FlwT3/1
  T6/1 -> [T6]
  [F7] -> FlwT7/1
  SOC8/1 -> [S8]
  [T7] -> T/7
  [R1] -> FlwR1/1
  T4/1 -> [T4]
  SOC6/1 -> [S6]
  [R5] -> FlwR5/1
  [F6] -> FlwT6/1
  [F1] -> FlwT1/1
  SOC/1 -> Bus Creator/1  "SOC"
  Bus Creator/1 -> State/1
  QT/1 -> Bus Selector/1
  Bus Selector/1 -> [F8], [F7], [F6], [F5], [F4], [F3], [F2], [F1]  "<FlwT>"
  Flow distribution to different modules/4(R4) -> [R4]
  Bus Selector/2 -> Flow distribution to different modules/1(<FlwR>)  "<FlwR>"
  Flow distribution to different modules/1(R1) -> [R1]
  Flow distribution to different modules/2(R2) -> [R2]
  Flow distribution to different modules/3(R3) -> [R3]
  Flow distribution to different modules/6(R6) -> [R6]
  Flow distribution to different modules/7(R7) -> [R7]
  Flow distribution to different modules/8(R8) -> [R8]
  Flow distribution to different modules/5(R5) -> [R5]
  connections:
  Module-5/LConn4 -- R56/LConn1
  Module-5/LConn3 -- R45/RConn1
  Module-7/LConn4 -- R78/LConn1
  T1/LConn1 -- Module-1/LConn2
  Ambient Temperature/LConn1 -- Module-8/RConn1 -- Module-7/RConn1 -- Module-6/RConn1 -- Module-5/RConn1 -- Module-4/RConn1 -- Module-3/RConn1 -- Module-2/RConn1 -- Module-1/RConn1
  R12/LConn1 -- Module-1/LConn4
  Module-3/LConn4 -- R34/LConn1
  Module-1/RConn2 -- FlwR1/RConn1
  Module-2/LConn3 -- R12/RConn1
  Module-3/LConn3 -- R23/RConn1
  Module-8/LConn4 -- neg/RConn1
  Module-1/LConn3 -- pos/RConn1
  SOC1/LConn1 -- Module-1/LConn1
  Module-8/LConn3 -- R78/RConn1
  Module-7/LConn3 -- R67/RConn1
  Module-6/LConn4 -- R67/LConn1
  Module-4/LConn3 -- R34/RConn1
  Module-2/LConn4 -- R23/LConn1
  Module-6/LConn3 -- R56/RConn1
  Module-1/RConn3 -- FlwT1/RConn1
  Module-4/LConn4 -- R45/LConn1
  SOC2/LConn1 -- Module-2/LConn1
  T2/LConn1 -- Module-2/LConn2
  Module-2/RConn3 -- FlwT2/RConn1
  Module-2/RConn2 -- FlwR2/RConn1
  Module-3/LConn2 -- T3/LConn1
  SOC3/LConn1 -- Module-3/LConn1
  Module-3/RConn3 -- FlwT3/RConn1
  FlwR3/RConn1 -- Module-3/RConn2
  Module-4/LConn2 -- T4/LConn1
  SOC4/LConn1 -- Module-4/LConn1
  FlwT4/RConn1 -- Module-4/RConn3
  FlwR4/RConn1 -- Module-4/RConn2
  Module-5/LConn1 -- SOC5/LConn1
  Module-5/LConn2 -- T5/LConn1
  FlwR5/RConn1 -- Module-5/RConn2
  Module-5/RConn3 -- FlwT5/RConn1
  Module-6/LConn1 -- SOC6/LConn1
  Module-6/LConn2 -- T6/LConn1
  FlwR6/RConn1 -- Module-6/RConn2
  FlwT6/RConn1 -- Module-6/RConn3
  Module-7/LConn1 -- SOC7/LConn1
  Module-7/LConn2 -- T7/LConn1
  FlwR7/RConn1 -- Module-7/RConn2
  FlwT7/RConn1 -- Module-7/RConn3
  Module-8/LConn1 -- SOC8/LConn1
  T8/LConn1 -- Module-8/LConn2
  FlwR8/RConn1 -- Module-8/RConn2
  FlwT8/RConn1 -- Module-8/RConn3
